simulink model "lw4"  (R2025a)
settings: Solver=VariableStepAuto  StartTime=0.0  StopTime=5  RelTol=1e-3
settings Model: Creator=user  LastModifiedBy=user

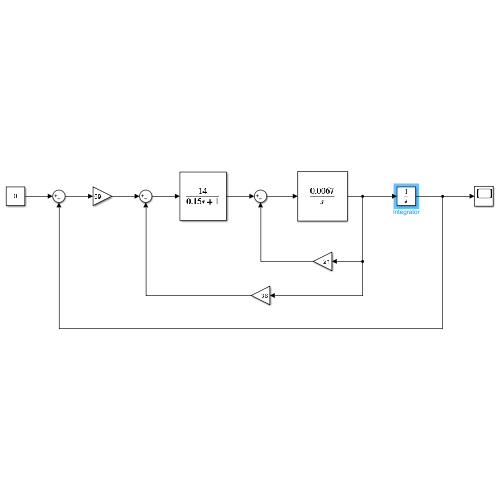
[thumbnail: Simulink's stored preview of the top-level diagram]
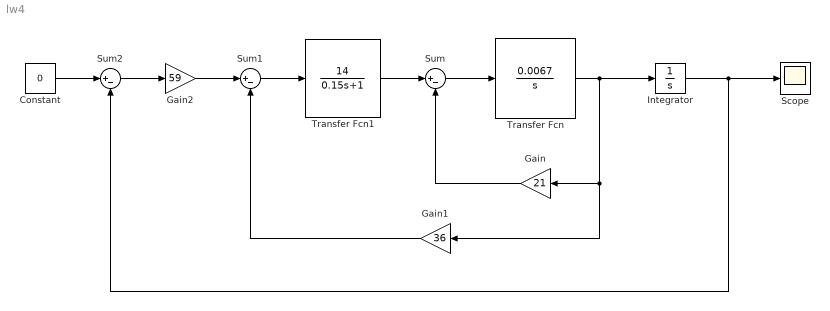
== system lw4 ==
  Constant : Constant  Value=0
  Gain : Gain  Gain=21
  Gain1 : Gain  Gain=36
  Gain2 : Gain  Gain=59
  Integrator : Integrator  InitialCondition=1
  Scope : Scope
      settings: ActiveDisplayYMinimum=-0.1811288520229159  ActiveDisplayYMaximum=1.1312365391136574
  Sum : Sum  Inputs=|+-
  Sum1 : Sum  Inputs=|+-
  Sum2 : Sum  Inputs=|+-
  Transfer Fcn : TransferFcn  Numerator=[0.0067]  Denominator=[1 0]
  Transfer Fcn1 : TransferFcn  Numerator=[14]  Denominator=[0.15 1]
  wires:
  Transfer Fcn/1 -> Integrator/1, Gain1/1, Gain/1
  Gain/1 -> Sum/2
  Transfer Fcn1/1 -> Sum/1
  Sum1/1 -> Transfer Fcn1/1
  Sum/1 -> Transfer Fcn/1
  Gain1/1 -> Sum1/2
  Gain2/1 -> Sum1/1
  Sum2/1 -> Gain2/1
  Constant/1 -> Sum2/1
  Integrator/1 -> Sum2/2, Scope/1
